simulink model "q4_b_simulink_PD"  (R2013a)
settings: Solver=ode45  StartTime=0.0  StopTime=100.0  RelTol=1e-3
values from neighbouring files (symbols this model uses):
  Kd = Kd_temp    [f.m]    (also in q4_b_PD.m = x1)
  Kp = Kp_temp    [f.m]    (also in q4_b_PD.m = x2)
settings Model: Creator=obrien94  LastModifiedBy=obrien94

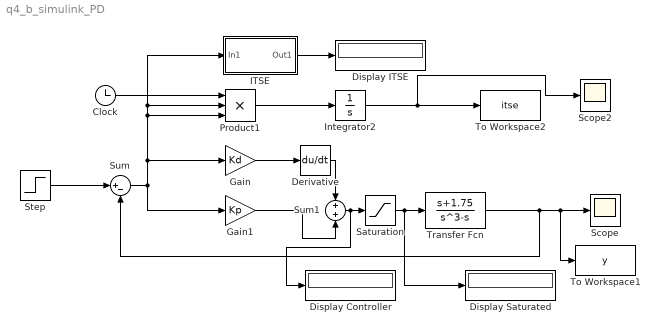
== system q4_b_simulink_PD ==
  Clock : Clock
  Derivative : Derivative
  Display Controller : Display
  Display ITSE : Display
  Display Saturated : Display
  Gain : Gain  Gain=Kd
  Gain1 : Gain  Gain=Kp
  ITSE : Subsystem
      mask help:
      | ISE performance index
      |
      | output = int (input)^2 dt
      mask Display:
      | disp('ITSE')
      | port_label('input',1,'e')
      | port_label('output',1,'itse')
  Integrator2 : Integrator
  Product1 : Product  Inputs=3
  Saturation : Saturate  UpperLimit=5  LowerLimit=-5
  Scope : Scope
  Scope2 : Scope
      settings: SaveName=ScopeData2
  Step : Step  SampleTime=0
  Sum : Sum  Inputs=|+-
  Sum1 : Sum
  To Workspace1 : ToWorkspace  VariableName=y  SampleTime=-1  SaveFormat=Timeseries
  To Workspace2 : ToWorkspace  VariableName=itse  SampleTime=-1
  Transfer Fcn : TransferFcn  Numerator=[1 1.75]  Denominator=[1 0 -1 0]
  wires:
  Step/1 -> Sum/1
  Sum/1 -> Product1/3, ITSE/1(In1), Product1/2, Gain/1, Gain1/1
  Transfer Fcn/1 -> Sum/2, To Workspace1/1, Scope/1
  Gain/1 -> Derivative/1
  Derivative/1 -> Sum1/1
  Sum1/1 -> Display Controller/1, Saturation/1
  Gain1/1 -> Sum1/2
  Integrator2/1 -> Scope2/1, To Workspace2/1
  Product1/1 -> Integrator2/1
  ITSE/1(Out1) -> Display ITSE/1
  Saturation/1 -> Display Saturated/1, Transfer Fcn/1
  Clock/1 -> Product1/1

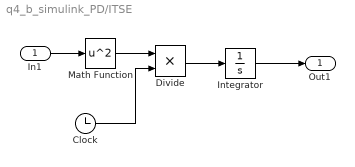
== system q4_b_simulink_PD/ITSE ==
  In1 : Inport
  Clock : Clock
  Divide : Product  Inputs=**
  Integrator : Integrator
  Math Function : Math  Operator=square  SaturateOnIntegerOverflow=on
  Out1 : Outport
  wires:
  Integrator/1 -> Out1/1
  In1/1 -> Math Function/1
  Divide/1 -> Integrator/1
  Math Function/1 -> Divide/1
  Clock/1 -> Divide/2
